simulink model "DC_Motor_Observer"  (R2023a)
settings: Solver=ode45  StartTime=0.0  StopTime=4  FixedStep=0.0001
values from neighbouring files (symbols this model uses):
  b = 0.0737    [DC_motor.m]
  C = 7*tf(numC,denC)    [DC_motor.m]
  J = 0.01    [DC_motor.m]
  K = 0.072    [DC_motor.m]
  La = 0.024    [DC_motor.m]
  Ra = 1.17    [DC_motor.m]
undefined symbols (not defined in the file or in its folder): A, B
settings Model: Creator=zaki  LastModifiedBy=nonyf
settings SolverCC: AlgebraicLoopSolver=TrustRegion
settings DebuggingCC: UnconnectedInputMsg=warning  UnconnectedOutputMsg=warning  UnconnectedLineMsg=warning
settings ModelReferenceCC: EnableRefExpFcnMdlSchedulingChecks=on
settings SFSimCC: CustomCodeUndefinedFunction=UseInterfaceOnly

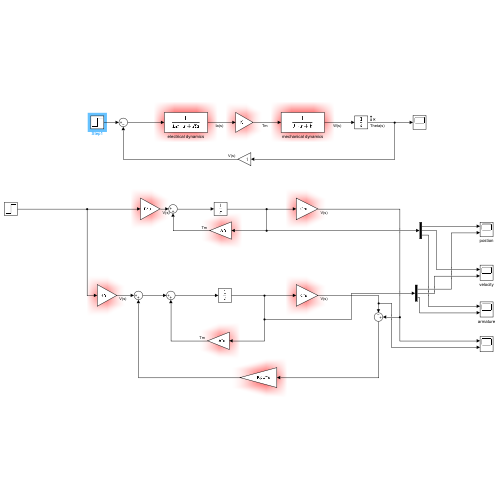
[thumbnail: Simulink's stored preview of the top-level diagram]
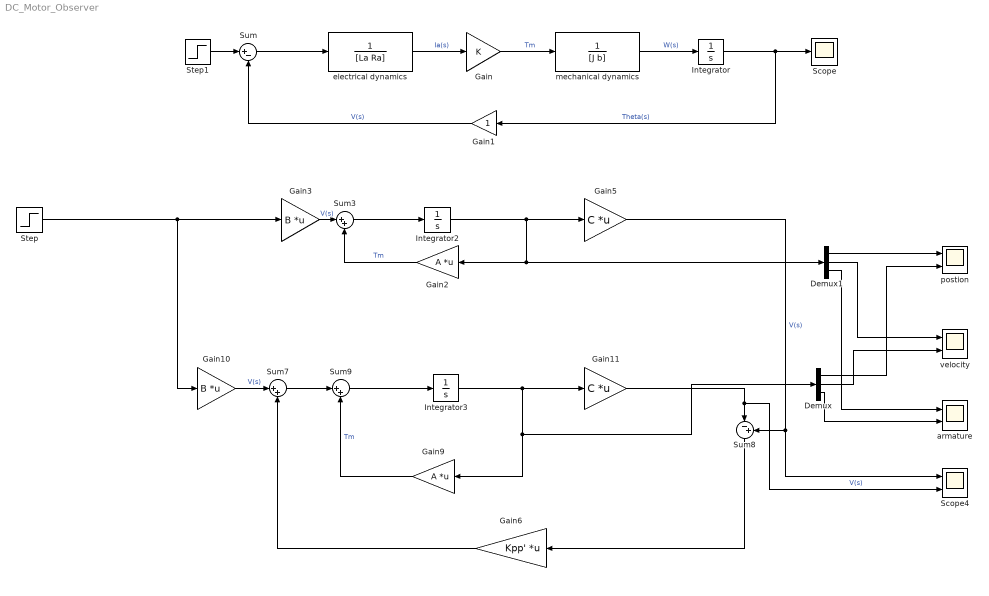
== system DC_Motor_Observer ==
  Demux : Demux  Outputs=3
  Demux1 : Demux  Outputs=3
  Gain : Gain  Gain=K
  Gain1 : Gain
  Gain10 : Gain  Gain=B  Multiplication=Matrix(K*u)
  Gain11 : Gain  Gain=C  Multiplication=Matrix(K*u)
  Gain2 : Gain  Gain=A  Multiplication=Matrix(K*u)
  Gain3 : Gain  Gain=B  Multiplication=Matrix(K*u)
  Gain5 : Gain  Gain=C  Multiplication=Matrix(K*u)
  Gain6 : Gain  Gain=Kpp'  Multiplication=Matrix(K*u)
  Gain9 : Gain  Gain=A  Multiplication=Matrix(K*u)
  Integrator : Integrator
  Integrator2 : Integrator
  Integrator3 : Integrator
  Scope : Scope
  Scope4 : Scope  NumInputPorts=2
  Step : Step  Time=0  After=pi/2  SampleTime=0
  Step1 : Step  Time=0  After=pi/2  SampleTime=0
  Sum : Sum  Inputs=|+-
  Sum3 : Sum  Inputs=|++
  Sum7 : Sum  Inputs=|++
  Sum8 : Sum  Inputs=|-+
  Sum9 : Sum  Inputs=|++
  armature : Scope  NumInputPorts=2
  electrical dynamics : TransferFcn  Denominator=[La Ra]
  mechanical dynamics : TransferFcn  Denominator=[J b]
  postion : Scope  NumInputPorts=2
  velocity : Scope  NumInputPorts=2
  wires:
  Sum/1 -> electrical dynamics/1
  electrical dynamics/1 -> Gain/1  "Ia(s)"
  Gain/1 -> mechanical dynamics/1  "Tm"
  mechanical dynamics/1 -> Integrator/1  "W(s)"
  Integrator/1 -> Gain1/1, Scope/1  "Theta(s)"
  Integrator2/1 -> Demux1/1, Gain2/1, Gain5/1
  Gain5/1 -> Scope4/1, Sum8/2  "V(s)"
  Gain2/1 -> Sum3/2  "Tm"
  Sum3/1 -> Integrator2/1
  Sum9/1 -> Integrator3/1
  Gain9/1 -> Sum9/2  "Tm"
  Integrator3/1 -> Demux/1, Gain9/1, Gain11/1
  Gain10/1 -> Sum7/1  "V(s)"
  Sum7/1 -> Sum9/1
  Gain11/1 -> Scope4/2, Sum8/1  "V(s)"
  Gain6/1 -> Sum7/2
  Sum8/1 -> Gain6/1
  Gain3/1 -> Sum3/1  "V(s)"
  Demux1/1 -> postion/1
  Demux/1 -> postion/2
  Demux1/2 -> velocity/1
  Demux/2 -> velocity/2
  Demux1/3 -> armature/1
  Demux/3 -> armature/2
  Step/1 -> Gain3/1, Gain10/1
  Gain1/1 -> Sum/2  "V(s)"
  Step1/1 -> Sum/1
